simulink library "optimizePathShapeRGP_ul"  (R2022a)
settings: Solver=VariableStepAuto  StartTime=0.0  StopTime=10.0  RelTol=1e-3
values from neighbouring files (symbols this model uses):
  hiLvlCtrl = block.DialogPrm(2).Data    [optimizeAltitude_Lvl2SFun.m]    (also in optimizeThrLenghtAndElevation_Lvl2sFun.m; optimizeTrajectory_Lvl2SFun.m)
  rgp = block.DialogPrm(1).Data    [optimizePathShapeRGP_Lvl2sFunc.m]    (also in optimizePathShapeRGP_init.m = GP.RecursiveGaussianProcess(hiLvlCtrl.RGPspatialCovFn,     h)
libraries: dspsigops x1
settings Model: Creator=Ayaz  LastModifiedBy=lhill8
settings SolverCC: AlgebraicLoopSolver=TrustRegion
settings DebuggingCC: UnconnectedInputMsg=warning  UnconnectedOutputMsg=warning  UnconnectedLineMsg=warning  SFMachineParentedDataDiag=warning

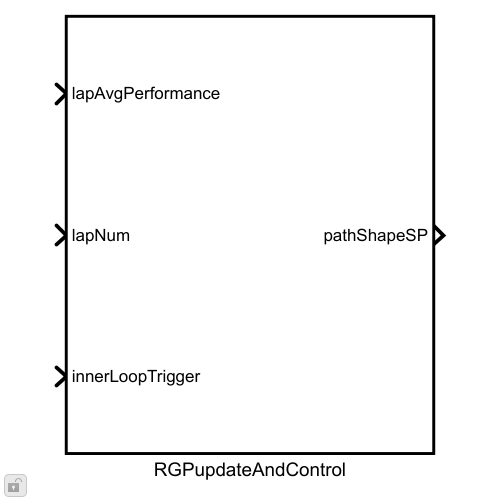
[thumbnail: Simulink's stored preview of the top-level diagram]
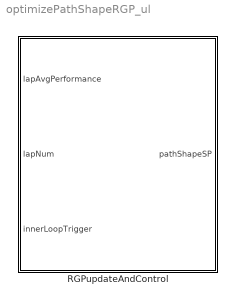
== system optimizePathShapeRGP_ul ==
  RGPupdateAndControl : Subsystem  TreatAsAtomicUnit=on  mask{hiLvlCtrl=hiLvlCtrl}
      mask prompts: hiLvlCtrl "High level controller object"
      mask init:
      | optimizePathShapeRGP_init

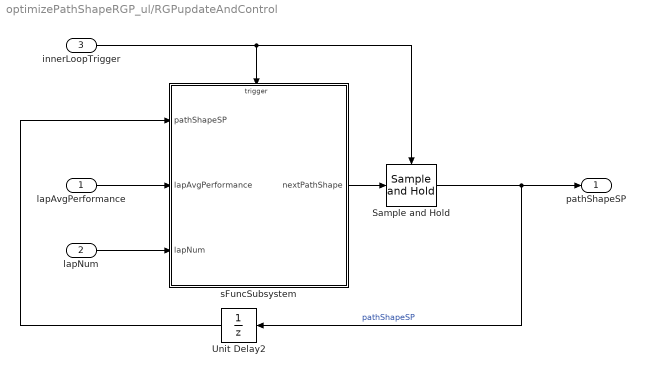
== system optimizePathShapeRGP_ul/RGPupdateAndControl ==
  lapAvgPerformance : Inport
  lapNum : Inport  Port=2
  innerLoopTrigger : Inport  Port=3
  Sample and Hold : dspsigops/Sample and Hold  trig=Rising edge  initCond=hiLvlCtrl.initPathShape  latchinput=off
  Unit Delay2 : UnitDelay  InitialCondition=hiLvlCtrl.initPathShape  SampleTime=-1  HasFrameUpgradeWarning=on
  sFuncSubsystem : Subsystem
  pathShapeSP : Outport
  wires:
  Sample and Hold/1 -> pathShapeSP/1, Unit Delay2/1  "pathShapeSP"
  lapAvgPerformance/1 -> sFuncSubsystem/2(lapAvgPerformance)
  lapNum/1 -> sFuncSubsystem/3(lapNum)
  sFuncSubsystem/1(nextPathShape) -> Sample and Hold/1
  Unit Delay2/1 -> sFuncSubsystem/1(pathShapeSP)
  innerLoopTrigger/1 -> Sample and Hold/Trigger, sFuncSubsystem/Trigger

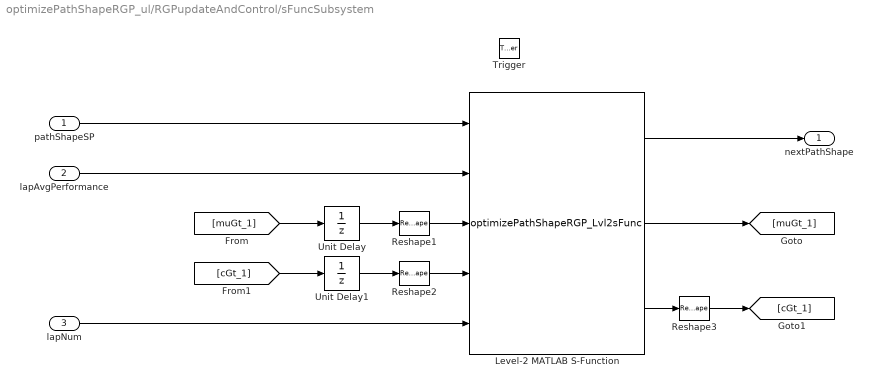
== system optimizePathShapeRGP_ul/RGPupdateAndControl/sFuncSubsystem ==
  pathShapeSP : Inport
  lapAvgPerformance : Inport  Port=2
  lapNum : Inport  Port=3
  Trigger : TriggerPort  VariantControl=Variant
  Level-2 MATLAB S-Function : M-S-Function  FunctionName=optimizePathShapeRGP_Lvl2sFunc  Parameters=rgp
  Reshape1 : Reshape  OutputDimensionality=Column vector (2-D)
  Reshape2 : Reshape  OutputDimensionality=Column vector (2-D)
  Reshape3 : Reshape  OutputDimensionality=Customize  OutputDimensions=length(rgp.meanFnVector)*[1,1]
  Unit Delay : UnitDelay  InitialCondition=rgp.meanFnVector  SampleTime=-1  HasFrameUpgradeWarning=on
  Unit Delay1 : UnitDelay  InitialCondition=rgp.spatialCovMat  SampleTime=-1  HasFrameUpgradeWarning=on
  nextPathShape : Outport
  wires:
  lapAvgPerformance/1 -> Level-2 MATLAB S-Function/2
  Unit Delay/1 -> Reshape1/1
  Reshape3/1 -> [cGt_1]
  Reshape2/1 -> Level-2 MATLAB S-Function/4
  pathShapeSP/1 -> Level-2 MATLAB S-Function/1
  Unit Delay1/1 -> Reshape2/1
  [muGt_1] -> Unit Delay/1
  Level-2 MATLAB S-Function/3 -> Reshape3/1
  Level-2 MATLAB S-Function/2 -> [muGt_1]
  Reshape1/1 -> Level-2 MATLAB S-Function/3
  [cGt_1] -> Unit Delay1/1
  lapNum/1 -> Level-2 MATLAB S-Function/5
  Level-2 MATLAB S-Function/1 -> nextPathShape/1
